simulink model "sim_mpc"  (R2025b)
settings: Solver=ode45  StartTime=0.0  StopTime=t_sim  MaxStep=0.001*Ts  MinStep=0.0001*Ts  RelTol=1e-3
undefined symbols (not defined in the file): C, md, rho, Ts
libraries: cstblocks x1
settings Model: Creator=davidecovolo  LastModifiedBy=davidecovolo
settings SolverCC: InitialStep=0.0001*Ts

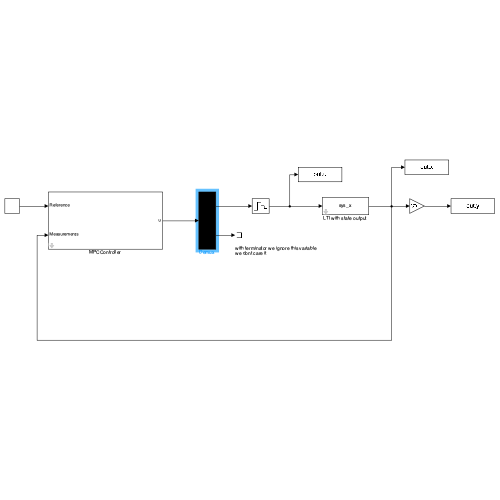
[thumbnail: Simulink's stored preview of the top-level diagram]
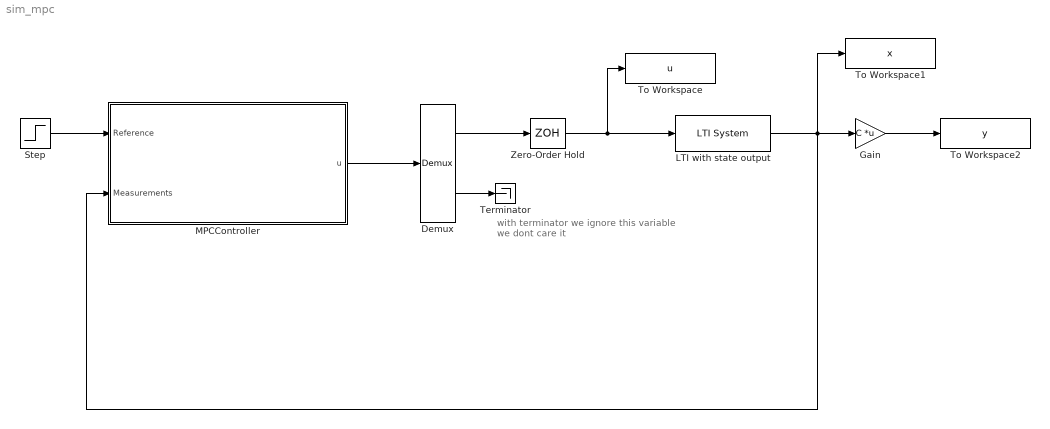
== system sim_mpc ==
  note: with terminator we ignore this variable
      | we dont care it
  Demux : Demux  Outputs=2
  Gain : Gain  Gain=C  Multiplication=Matrix(K*u)
  LTI with state output : cstblocks/LTI System  sys=sys_x  IC=[]  PadeOrder=0
  MPCController : Subsystem  mask{md=md}
      mask prompts: md "MPCData"
  Step : Step  Time=0  After=rho  SampleTime=0
  Terminator : Terminator
  To Workspace : ToWorkspace  VariableName=u  SaveFormat=Timeseries  SampleTime=Ts
  To Workspace1 : ToWorkspace  VariableName=x  SaveFormat=Timeseries  SampleTime=Ts
  To Workspace2 : ToWorkspace  VariableName=y  SaveFormat=Timeseries  SampleTime=Ts
  Zero-Order Hold : ZeroOrderHold  SampleTime=Ts
  wires:
  MPCController/1(u) -> Demux/1
  Demux/1 -> Zero-Order Hold/1
  Zero-Order Hold/1 -> To Workspace/1, LTI with state output/1
  LTI with state output/1 -> To Workspace1/1, MPCController/2(Measurements), Gain/1
  Gain/1 -> To Workspace2/1
  Step/1 -> MPCController/1(Reference)
  Demux/2 -> Terminator/1

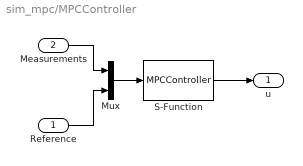
== system sim_mpc/MPCController ==
  Reference : Inport
  Measurements : Inport  Port=2
  Mux : Mux  Inputs=2
  S-Function : S-Function  FunctionName=MPCController  Parameters=md  SFunctionDeploymentMode=off  EnableBusSupport=off
  u : Outport
  wires:
  Mux/1 -> S-Function/1
  Measurements/1 -> Mux/1
  Reference/1 -> Mux/2
  S-Function/1 -> u/1
